simulink model "ukol5_model"  (R2012b)
settings: Solver=ode45  StartTime=0.0  StopTime=10.0  RelTol=1e-3
settings Model: Creator=student  LastModifiedBy=student

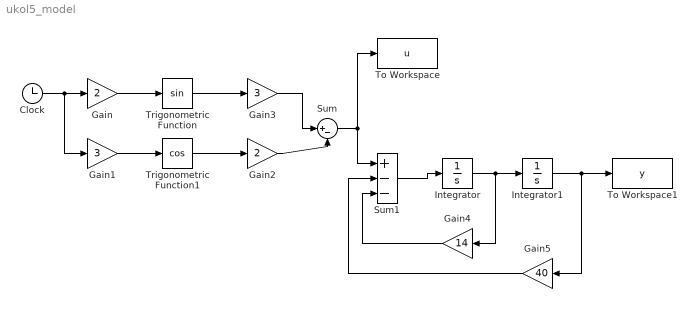
== system ukol5_model ==
  Clock : Clock
  Gain : Gain  Gain=2
  Gain1 : Gain  Gain=3
  Gain2 : Gain  Gain=2
  Gain3 : Gain  Gain=3
  Gain4 : Gain  Gain=14
  Gain5 : Gain  Gain=40
  Integrator : Integrator
  Integrator1 : Integrator
  Sum : Sum  Inputs=|+-
  Sum1 : Sum  Inputs=+--
  To Workspace : ToWorkspace  VariableName=u  SampleTime=-1  SaveFormat=Structure With Time
  To Workspace1 : ToWorkspace  VariableName=y  SampleTime=-1  SaveFormat=Structure With Time
  Trigonometric Function : Trigonometry
  Trigonometric Function1 : Trigonometry  Operator=cos
  wires:
  Clock/1 -> Gain1/1, Gain/1
  Gain/1 -> Trigonometric Function/1
  Gain1/1 -> Trigonometric Function1/1
  Trigonometric Function/1 -> Gain3/1
  Trigonometric Function1/1 -> Gain2/1
  Gain3/1 -> Sum/1
  Gain2/1 -> Sum/2
  Sum/1 -> To Workspace/1, Sum1/1
  Sum1/1 -> Integrator/1
  Integrator/1 -> Gain4/1, Integrator1/1
  Integrator1/1 -> Gain5/1, To Workspace1/1
  Gain4/1 -> Sum1/3
  Gain5/1 -> Sum1/2
